simulink model "AMCLIB_FW_BAM"  (Simulink 9.3)
settings: Solver=VariableStepAuto  StartTime=0.0  StopTime=10.0  RelTol=1e-3
settings Model: Creator=nxa18952  LastModifiedBy=nxa18952
settings DataIOCC: SaveFormat=Dataset  SignalLoggingSaveFormat=Dataset  ReturnWorkspaceOutputs=on
settings OptimizationCC: LifeSpan=auto
settings DebuggingCC: UnderspecifiedInitializationDetection=Simplified  MergeDetectMultiDrivingBlocksExec=error  FcnCallInpInsideContextMsg=error  SFUnexpectedBacktrackingDiag=error  SFNoUnconditionalDefaultTransitionDiag=error  SFExecutionAtInitializationDiag=warning  ArithmeticOperatorsInVariantConditions=error
settings HardwareCC: ProdBitPerPointer=64  ProdBitPerSizeT=64  ProdBitPerPtrDiffT=64  ProdLargestAtomicFloat=Float  ProdIntDivRoundTo=Zero  ProdEndianess=LittleEndian  ProdWordSize=64  ProdHWDeviceType=Intel->x86-64 (Windows64)
settings ModelReferenceCC: PropagateSignalLabelsOutOfModel=on
settings SFSimCC: SimUseLocalCustomCode=on
settings RTWCC: RTWUseLocalCustomCode=on
settings CodeAppCC: StateflowObjectComments=off
settings GRTTargetCC: TargetLangStandard=C99 (ISO)  CombineOutputUpdateFcns=on  GRTInterface=off
settings ConfigComp: CovMetricSettings=dwe  CovHtmlReporting=off  CovSaveCumulativeToWorkspaceVar=off  CovSaveSingleToWorkspaceVar=off  CovExternalEMLEnable=on

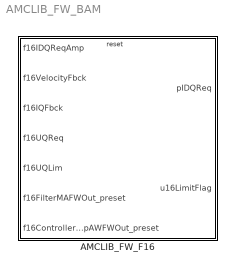
== system AMCLIB_FW_BAM ==
  AMCLIB_FW_F16 : Subsystem  TreatAsAtomicUnit=on  mask(AMCLIB_FW_F16){showStates=Hide (faster execution), resetStatesEnable=Pre-set according to the first set of inputs after reset, showDebugOutputs=Hide, u16NSamples=0, f16PropGain=0, f16IntegGain=0, s16PropGainShift=0, s16IntegGainShift=0, f16LowerLimit=0, f16UpperLimit=0}
      mask prompts: showStates "Show internal states"; resetStatesEnable "Internal state after reset"; showDebugOutputs "Show debugging outputs"; u16NSamples "u16NSamples (GDFLIB_FilterMA - recalculated smoothing factor)"; f16PropGain "f16PropGain (GFLIB_ControllerPIpAW - proportional gain)"; f16IntegGain "f16IntegGain (GFLIB_ControllerPIpAW - integral gain)"; s16PropGainShift "s16PropGainShift (GFLIB_ControllerPIpAW - scaling bitwise shift applied to the proportional gain)"; s16IntegGainShift "s16IntegGainShift (GFLIB_ControllerPIpAW - scaling bitwise shift applied to the integral gain)"; f16LowerLimit "f16LowerLimit (GFLIB_ControllerPIpAW - lower limit)"; f16UpperLimit "f16UpperLimit (GFLIB_ControllerPIpAW - upper limit)"
      mask help: Field Weakening controller for the PMSM field-oriented control algorithm in 16-bit fixed-point fractional implementation. This block supports re-initialization of the internal state during simulation. If the block is reset, the output of the MA filter and PI controller will be aligned with the inputs f16FilterMAFWOut_preset and f16ControllerPIpAWFWOut_preset. Refer to the AMMCLIB User's Guide for further details.
      mask init:
      | if ~evalin('base','exist(''tS8'',''var'')')
      |   if (2 ~= exist('SWLIBS_Typedefs.mat','file'))
      |       error('File SWLIBS_Typedefs.mat is not on the Matlab path. Please add the AMMCLIB "bam" folder in the Matlab Search Path.');
      |   else
      |       evalin('base', 'load(''SWLIBS_Typedefs.mat'')');
      |   end
      | end
      | if showStates == 1
      |     % hidden state variables
      |     if strcmp(get_param([gcb '/u16NSamples'], 'BlockType'), 'Inport')
      |         posblk = get_param(gcb, 'Position');
      | 
      |         pos = get_param(    [gcb, '/u16NSamples'], 'Position');
      |         orient = get_param( [gcb, '/u16NSamples'], 'Orientation');
      |         delete_block(       [gcb, '/u16NSamples']);
      |         add_block('built-in/Ground', [gcb, '/u16NSamples'], 'Position', pos, 'Orientation', orient);
      | 
      |         pos = get_param(    [gcb, '/f16PropGain'], 'Position');
      |         orient = get_param( [gcb, '/f16PropGain'], 'Orientation');
      |         delete_block(       [gcb, '/f16PropGain']);
      |         add_block('built-in/Ground', [gcb, '/f16PropGain'], 'Position', pos, 'Orientation', orient);
      | 
      |         pos = get_param(    [gcb, '/f16IntegGain'], 'Position');
      |         orient = get_param( [gcb, '/f16IntegGain'], 'Orientation');
      |         delete_block(       [gcb, '/f16IntegGain']);
      |         add_block('built-in/Ground', [gcb, '/f16IntegGain'], 'Position', pos, 'Orientation', orient);
      | 
      |         pos = get_param(    [gcb, '/s16PropGainShift'], 'Position');
      |         orient = get_param( [gcb, '/s16PropGainShift'], 'Orientation');
      |         delete_block(       [gcb, '/s16PropGainShift']);
      |         add_block('built-in/Ground', [gcb, '/s16PropGainShift'], 'Position', pos, 'Orientation', orient);
      | 
      |         pos = get_param(    [gcb, '/s16IntegGainShift'], 'Position');
      |         orient = get_param( [gcb, '/s16IntegGainShift'], 'Orientation');
      |         delete_block(       [gcb, '/s16IntegGainShift']);
      |         add_block('built-in/Ground', [gcb, '/s16IntegGainShift'], 'Position', pos, 'Orientation', orient);
      | 
      |         pos = get_param(    [gcb, '/f16LowerLimit'], 'Position');
      |         orient = get_param( [gcb, '/f16LowerLimit'], 'Orientation');
      |         delete_block(       [gcb, '/f16LowerLimit']);
      |         add_block('built-in/Ground', [gcb, '/f16LowerLimit'], 'Position', pos, 'Orientation', orient);
      | 
      |         pos = get_param(    [gcb, '/f16UpperLimit'], 'Position');
      |         orient = get_param( [gcb, '/f16UpperLimit'], 'Orientation');
      |         delete_block(       [gcb, '/f16UpperLimit']);
      |         add_block('built-in/Ground', [gcb, '/f16UpperLimit'], 'Position', pos, 'Orientation', orient);
      | 
      |         pos = get_param(    [gcb, '/f16IQReqK_1'], 'Position');
      |         orient = get_param( [gcb, '/f16IQReqK_1'], 'Orientation');
      |         delete_block(       [gcb, '/f16IQReqK_1']);
      |         add_block('built-in/Ground', [gcb, '/f16IQReqK_1'], 'Position', pos, 'Orientation', orient);
      | 
      |         pos = get_param(    [gcb, '/f32Acc'], 'Position');
      |         orient = get_param( [gcb, '/f32Acc'], 'Orientation');
      |         delete_block(       [gcb, '/f32Acc']);
      |         add_block('built-in/Ground', [gcb, '/f32Acc'], 'Position', pos, 'Orientation', orient);
      | 
      |         pos = get_param(    [gcb, '/f32IntegPartK_1'], 'Position');
      |         orient = get_param( [gcb, '/f32IntegPartK_1'], 'Orientation');
      |         delete_block(       [gcb, '/f32IntegPartK_1']);
      |         add_block('built-in/Ground', [gcb, '/f32IntegPartK_1'], 'Position', pos, 'Orientation', orient);
      | 
      |         pos = get_param(    [gcb, '/f16InK_1'], 'Position');
      |         orient = get_param( [gcb, '/f16InK_1'], 'Orientation');
      |         delete_block(       [gcb, '/f16InK_1']);
      |         add_block('built-in/Ground', [gcb, '/f16InK_1'], 'Position', pos, 'Orientation', orient);
      | 
      | 
      |         pos = get_param(    [gcb '/f32Acc_Out'], 'Position');
      |         orient = get_param( [gcb '/f32Acc_Out'], 'Orientation');
      |         delete_block(       [gcb '/f32Acc_Out']);
      |         add_block('built-in/Terminator', [gcb '/f32Acc_Out'], 'Position', pos, 'Orientation', orient);
      | 
      |         pos = get_param(    [gcb '/f32IntegPartK_1_Out'], 'Position');
      |         orient = get_param( [gcb '/f32IntegPartK_1_Out'], 'Orientation');
      |         delete_block(       [gcb '/f32IntegPartK_1_Out']);
      |         add_block('built-in/Terminator', [gcb '/f32IntegPartK_1_Out'], 'Position', pos, 'Orientation', orient);
      | 
      |         pos = get_param(    [gcb '/f16InK_1_Out'], 'Position');
      |         orient = get_param( [gcb '/f16InK_1_Out'], 'Orientation');
      |         delete_block(       [gcb '/f16InK_1_Out']);
      |         add_block('built-in/Terminator', [gcb '/f16InK_1_Out'], 'Position', pos, 'Orientation', orient);
      | 
      | 
      |         if strcmp(get_param([gcb '/f16IQErrSign'], 'BlockType'), 'Outport')
      |             pos = get_param(    [gcb '/f16IQErrSign'], 'Position');
      |             orient = get_param( [gcb '/f16IQErrSign'], 'Orientation');
      |             delete_block(       [gcb '/f16IQErrSign']);
      |             add_block('built-in/Terminator', [gcb '/f16IQErrSign'], 'Position', pos, 'Orientation', orient);
      | 
      |             pos = get_param(    [gcb '/f16IQErr'], 'Position');
      |             orient = get_param( [gcb '/f16IQErr'], 'Orientation');
      |             delete_block(       [gcb '/f16IQErr']);
      |             add_block('built-in/Terminator', [gcb '/f16IQErr'], 'Position', pos, 'Orientation', orient);
      | 
      |             pos = get_param(    [gcb '/f16FWErr'], 'Position');
      |             orient = get_param( [gcb '/f16FWErr'], 'Orientation');
      |             delete_block(       [gcb '/f16FWErr']);
      |             add_block('built-in/Terminator', [gcb '/f16FWErr'], 'Position', pos, 'Orientation', orient);
      | 
      |             pos = get_param(    [gcb '/f16UQErr'], 'Position');
      |             orient = get_param( [gcb '/f16UQErr'], 'Orientation');
      |             delete_block(       [gcb '/f16UQErr']);
      |             add_block('built-in/Terminator', [gcb '/f16UQErr'], 'Position', pos, 'Orientation', orient);
      | 
      |             pos = get_param(    [gcb '/f16FWErrFilt'], 'Position');
      |             orient = get_param( [gcb '/f16FWErrFilt'], 'Orientation');
      |             delete_block(       [gcb '/f16FWErrFilt']);
      |             add_block('built-in/Terminator', [gcb '/f16FWErrFilt'], 'Position', pos, 'Orientation', orient);
      | 
      |             pos = get_param(    [gcb '/f16FWAngle'], 'Position');
      |             orient = get_param( [gcb '/f16FWAngle'], 'Orientation');
      |             delete_block(       [gcb '/f16FWAngle']);
      |             add_block('built-in/Terminator', [gcb '/f16FWAngle'], 'Position', pos, 'Orientation', orient);
      | 
      |             pos = get_param(    [gcb '/f16FWSin'], 'Position');
      |             orient = get_param( [gcb '/f16FWSin'], 'Orientation');
      |             delete_block(       [gcb '/f16FWSin']);
      |             add_block('built-in/Terminator', [gcb '/f16FWSin'], 'Position', pos, 'Orientation', orient);
      | 
      |             pos = get_param(    [gcb '/f16FWCos'], 'Position');
      |             orient = get_param( [gcb '/f16FWCos'], 'Orientation');
      |             delete_block(       [gcb '/f16FWCos']);
      |             add_block('built-in/Terminator', [gcb '/f16FWCos'], 'Position', pos, 'Orientation', orient);
      | 
      |         end
      | 
      |         set_param([gcb '/f16IDQReqAmp'], 'Port', '1');
      |         set_param([gcb '/f16VelocityFbck'], 'Port', '2');
      |         set_param([gcb '/f16IQFbck'], 'Port', '3');
      |         set_param([gcb '/f16UQReq'], 'Port', '4');
      |         set_param([gcb '/f16UQLim'], 'Port', '5');
      |         set_param([gcb '/f16FilterMAFWOut_preset'], 'Port', '6');
      |         set_param([gcb '/f16ControllerPIpAWFWOut_preset'], 'Port', '7');
      | 
      |         set_param([gcb '/pIDQReq'], 'Port', '1');
      |         set_param([gcb '/u16LimitFlag'], 'Port', '2');
      | 
      |         set_param(gcb,'MaskEnables',{'on','on','off','on','on','on','on','on','on','on'});
      | 
      |         if (posblk(4) - posblk(2)) > 200
      |           height = 200;
      |           set_param(gcb,'Position',[posblk(1), posblk(2), posblk(3), posblk(2)+height])
      |         end
      |     end
      | else
      |     % shown state variables
      |     if strcmp(get_param([gcb '/u16NSamples'], 'BlockType'), 'Ground')
      |         posblk = get_param(gcb, 'Position');
      | 
      |         pos = get_param(    [gcb, '/u16NSamples'], 'Position');
      |         orient = get_param( [gcb, '/u16NSamples'], 'Orientation');
      |         delete_block(       [gcb, '/u16NSamples']);
      |         add_block('built-in/Inport', [gcb, '/u16NSamples'], 'Position', pos, 'Orientation', orient, 'OutDataTypeStr', 'uint16');
      | 
      |         pos = get_param(    [gcb, '/f16PropGain'], 'Position');
      |         orient = get_param( [gcb, '/f16PropGain'], 'Orientation');
      |         delete_block(       [gcb, '/f16PropGain']);
      |         add_block('built-in/Inport', [gcb, '/f16PropGain'], 'Position', pos, 'Orientation', orient, 'OutDataTypeStr', 'int16');
      | 
      |         pos = get_param(    [gcb, '/f16IntegGain'], 'Position');
      |         orient = get_param( [gcb, '/f16IntegGain'], 'Orientation');
      |         delete_block(       [gcb, '/f16IntegGain']);
      |         add_block('built-in/Inport', [gcb, '/f16IntegGain'], 'Position', pos, 'Orientation', orient, 'OutDataTypeStr', 'int16');
      | 
      |         pos = get_param(    [gcb, '/s16PropGainShift'], 'Position');
      |         orient = get_param( [gcb, '/s16PropGainShift'], 'Orientation');
      |         delete_block(       [gcb, '/s16PropGainShift']);
      |         add_block('built-in/Inport', [gcb, '/s16PropGainShift'], 'Position', pos, 'Orientation', orient, 'OutDataTypeStr', 'int16');
      | 
      |         pos = get_param(    [gcb, '/s16IntegGainShift'], 'Position');
      |         orient = get_param( [gcb, '/s16IntegGainShift'], 'Orientation');
      |         delete_block(       [gcb, '/s16IntegGainShift']);
      |         add_block('built-in/Inport', [gcb, '/s16IntegGainShift'], 'Position', pos, 'Orientation', orient, 'OutDataTypeStr', 'int16');
      | 
      |         pos = get_param(    [gcb, '/f16LowerLimit'], 'Position');
      |         orient = get_param( [gcb, '/f16LowerLimit'], 'Orientation');
      |         delete_block(       [gcb, '/f16LowerLimit']);
      |         add_block('built-in/Inport', [gcb, '/f16LowerLimit'], 'Position', pos, 'Orientation', orient, 'OutDataTypeStr', 'int16');
      | 
      |         pos = get_param(    [gcb, '/f16UpperLimit'], 'Position');
      |         orient = get_param( [gcb, '/f16UpperLimit'], 'Orientation');
      |         delete_block(       [gcb, '/f16UpperLimit']);
      |         add_block('built-in/Inport', [gcb, '/f16UpperLimit'], 'Position', pos, 'Orientation', orient, 'OutDataTypeStr', 'int16');
      | 
      |         pos = get_param(    [gcb, '/f16IQReqK_1'], 'Position');
      |         orient = get_param( [gcb, '/f16IQReqK_1'], 'Orientation');
      |         delete_block(       [gcb, '/f16IQReqK_1']);
      |         add_block('built-in/Inport', [gcb, '/f16IQReqK_1'], 'Position', pos, 'Orientation', orient, 'OutDataTypeStr', 'int16');
      | 
      |         pos = get_param(    [gcb, '/f32Acc'], 'Position');
      |         orient = get_param( [gcb, '/f32Acc'], 'Orientation');
      |         delete_block(       [gcb, '/f32Acc']);
      |         add_block('built-in/Inport', [gcb, '/f32Acc'], 'Position', pos, 'Orientation', orient, 'OutDataTypeStr', 'int32');
      | 
      |         pos = get_param(    [gcb, '/f32IntegPartK_1'], 'Position');
      |         orient = get_param( [gcb, '/f32IntegPartK_1'], 'Orientation');
      |         delete_block(       [gcb, '/f32IntegPartK_1']);
      |         add_block('built-in/Inport', [gcb, '/f32IntegPartK_1'], 'Position', pos, 'Orientation', orient, 'OutDataTypeStr', 'int32');
      | 
      |         pos = get_param(    [gcb, '/f16InK_1'], 'Position');
      |         orient = get_param( [gcb, '/f16InK_1'], 'Orientation');
      |         delete_block(       [gcb, '/f16InK_1']);
      |         add_block('built-in/Inport', [gcb, '/f16InK_1'], 'Position', pos, 'Orientation', orient, 'OutDataTypeStr', 'int16');
      | 
      | 
      |         pos = get_param(    [gcb '/f32Acc_Out'], 'Position');
      |         orient = get_param( [gcb '/f32Acc_Out'], 'Orientation');
      |         delete_block(       [gcb '/f32Acc_Out']);
      |         add_block('built-in/Outport', [gcb '/f32Acc_Out'], 'Position', pos, 'Orientation', orient);
      | 
      |         pos = get_param(    [gcb '/f32IntegPartK_1_Out'], 'Position');
      |         orient = get_param( [gcb '/f32IntegPartK_1_Out'], 'Orientation');
      |         delete_block(       [gcb '/f32IntegPartK_1_Out']);
      |         add_block('built-in/Outport', [gcb '/f32IntegPartK_1_Out'], 'Position', pos, 'Orientation', orient);
      | 
      |         pos = get_param(    [gcb '/f16InK_1_Out'], 'Position');
      |         orient = get_param( [gcb '/f16InK_1_Out'], 'Orientation');
      |         delete_block(       [gcb '/f16InK_1_Out']);
      |         add_block('built-in/Outport', [gcb '/f16InK_1_Out'], 'Position', pos, 'Orientation', orient);
      | 
      | 
      |         if (showDebugOutputs == 2) && (strcmp(get_param([gcb '/f16IQErrSign'], 'BlockType'), 'Terminator'))
      |             pos = get_param(    [gcb '/f16IQErrSign'], 'Position');
      |             orient = get_param( [gcb '/f16IQErrSign'], 'Orientation');
      |             delete_block(       [gcb '/f16IQErrSign']);
      |             add_block('built-in/Outport', [gcb '/f16IQErrSign'], 'Position', pos, 'Orientation', orient);
      | 
      |             pos = get_param(    [gcb '/f16IQErr'], 'Position');
      |             orient = get_param( [gcb '/f16IQErr'], 'Orientation');
      |             delete_block(       [gcb '/f16IQErr']);
      |             add_block('built-in/Outport', [gcb '/f16IQErr'], 'Position', pos, 'Orientation', orient);
      | 
      |             pos = get_param(    [gcb '/f16FWErr'], 'Position');
      |             orient = get_param( [gcb '/f16FWErr'], 'Orientation');
      |             delete_block(       [gcb '/f16FWErr']);
      |             add_block('built-in/Outport', [gcb '/f16FWErr'], 'Position', pos, 'Orientation', orient);
      | 
      |             pos = get_param(    [gcb '/f16UQErr'], 'Position');
      |             orient = get_param( [gcb '/f16UQErr'], 'Orientation');
      |             delete_block(       [gcb '/f16UQErr']);
      |             add_block('built-in/Outport', [gcb '/f16UQErr'], 'Position', pos, 'Orientation', orient);
      | 
      |             pos = get_param(    [gcb '/f16FWErrFilt'], 'Position');
      |             orient = get_param( [gcb '/f16FWErrFilt'], 'Orientation');
      |             delete_block(       [gcb '/f16FWErrFilt']);
      |             add_block('built-in/Outport', [gcb '/f16FWErrFilt'], 'Position', pos, 'Orientation', orient);
      | 
      |             pos = get_param(    [gcb '/f16FWAngle'], 'Position');
      |             orient = get_param( [gcb '/f16FWAngle'], 'Orientation');
      |             delete_block(       [gcb '/f16FWAngle']);
      |             add_block('built-in/Outport', [gcb '/f16FWAngle'], 'Position', pos, 'Orientation', orient);
      | 
      |             pos = get_param(    [gcb '/f16FWSin'], 'Position');
      |             orient = get_param( [gcb '/f16FWSin'], 'Orientation');
      |             delete_block(       [gcb '/f16FWSin']);
      |             add_block('built-in/Outport', [gcb '/f16FWSin'], 'Position', pos, 'Orientation', orient);
      | 
      |             pos = get_param(    [gcb '/f16FWCos'], 'Position');
      |             orient = get_param( [gcb '/f16FWCos'], 'Orientation');
      |             delete_block(       [gcb '/f16FWCos']);
      |             add_block('built-in/Outport', [gcb '/f16FWCos'], 'Position', pos, 'Orientation', orient);
      | 
      |         end
      | 
      |         set_param([gcb '/f16IDQReqAmp'], 'Port', '1');
      |         set_param([gcb '/f16VelocityFbck'], 'Port', '2');
      |         set_param([gcb '/f16IQFbck'], 'Port', '3');
      |         set_param([gcb '/f16UQReq'], 'Port', '4');
      |         set_param([gcb '/f16UQLim'], 'Port', '5');
      |         set_param([gcb '/f16FilterMAFWOut_preset'], 'Port', '6');
      |         set_param([gcb '/f16ControllerPIpAWFWOut_preset'], 'Port', '7');
      |         set_param([gcb '/u16NSamples'], 'Port', '8');
      |         set_param([gcb '/f16PropGain'], 'Port', '9');
      |         set_param([gcb '/f16IntegGain'], 'Port', '10');
      |         set_param([gcb '/s16PropGainShift'], 'Port', '11');
      |         set_param([gcb '/s16IntegGainShift'], 'Port', '12');
      |         set_param([gcb '/f16LowerLimit'], 'Port', '13');
      |         set_param([gcb '/f16UpperLimit'], 'Port', '14');
      |         set_param([gcb '/f16IQReqK_1'], 'Port', '15');
      |         set_param([gcb '/f32Acc'], 'Port', '16');
      |         set_param([gcb '/f32IntegPartK_1'], 'Port', '17');
      |         set_param([gcb '/f16InK_1'], 'Port', '18');
      | 
      |         if (showDebugOutputs == 2)
      |             set_param([gcb '/pIDQReq'], 'Port', '1');
      |             set_param([gcb '/u16LimitFlag'], 'Port', '2');
      |             set_param([gcb '/f16IQErrSign'], 'Port', '3');
      |             set_param([gcb '/f16IQErr'], 'Port', '4');
      |             set_param([gcb '/f16FWErr'], 'Port', '5');
      |             set_param([gcb '/f16UQErr'], 'Port', '6');
      |             set_param([gcb '/f16FWErrFilt'], 'Port', '7');
      |             set_param([gcb '/f16FWAngle'], 'Port', '8');
      |             set_param([gcb '/f16FWSin'], 'Port', '9');
      |             set_param([gcb '/f16FWCos'], 'Port', '10');
      |             set_param([gcb '/f32Acc_Out'], 'Port', '11');
      |             set_param([gcb '/f32IntegPartK_1_Out'], 'Port', '12');
      |             set_param([gcb '/f16InK_1_Out'], 'Port', '13');
      |         else
      |             set_param([gcb '/pIDQReq'], 'Port', '1');
      |             set_param([gcb '/u16LimitFlag'], 'Port', '2');
      |             set_param([gcb '/f32Acc_Out'], 'Port', '3');
      |             set_param([gcb '/f32IntegPartK_1_Out'], 'Port', '4');
      |             set_param([gcb '/f16InK_1_Out'], 'Port', '5');
      |         end
      | 
      |         set_param(gcb,'MaskEnables',{'on','on','on','off','off','off','off','off','off','off'});
      | 
      |         if (posblk(4) - posblk(2)) < 475
      |           height = 475;
      |           set_param(gcb,'Position',[posblk(1), posblk(2), posblk(3), posblk(2)+height])
      |         end
      |     else
      |         if (showDebugOutputs == 2) && (strcmp(get_param([gcb '/f16IQErrSign'], 'BlockType'), 'Terminator'))
      |             % shown debugging outputs
      |             pos = get_param(    [gcb '/f16IQErrSign'], 'Position');
      |             orient = get_param( [gcb '/f16IQErrSign'], 'Orientation');
      |             delete_block(       [gcb '/f16IQErrSign']);
      |             add_block('built-in/Outport', [gcb '/f16IQErrSign'], 'Position', pos, 'Orientation', orient);
      | 
      |             pos = get_param(    [gcb '/f16IQErr'], 'Position');
      |             orient = get_param( [gcb '/f16IQErr'], 'Orientation');
      |             delete_block(       [gcb '/f16IQErr']);
      |             add_block('built-in/Outport', [gcb '/f16IQErr'], 'Position', pos, 'Orientation', orient);
      | 
      |             pos = get_param(    [gcb '/f16FWErr'], 'Position');
      |             orient = get_param( [gcb '/f16FWErr'], 'Orientation');
      |             delete_block(       [gcb '/f16FWErr']);
      |             add_block('built-in/Outport', [gcb '/f16FWErr'], 'Position', pos, 'Orientation', orient);
      | 
      |             pos = get_param(    [gcb '/f16UQErr'], 'Position');
      |             orient = get_param( [gcb '/f16UQErr'], 'Orientation');
      |             delete_block(       [gcb '/f16UQErr']);
      |             add_block('built-in/Outport', [gcb '/f16UQErr'], 'Position', pos, 'Orientation', orient);
      | 
      |             pos = get_param(    [gcb '/f16FWErrFilt'], 'Position');
      |             orient = get_param( [gcb '/f16FWErrFilt'], 'Orientation');
      |             delete_block(       [gcb '/f16FWErrFilt']);
      |             add_block('built-in/Outport', [gcb '/f16FWErrFilt'], 'Position', pos, 'Orientation', orient);
      | 
      |             pos = get_param(    [gcb '/f16FWAngle'], 'Position');
      |             orient = get_param( [gcb '/f16FWAngle'], 'Orientation');
      |             delete_block(       [gcb '/f16FWAngle']);
      |             add_block('built-in/Outport', [gcb '/f16FWAngle'], 'Position', pos, 'Orientation', orient);
      | 
      |             pos = get_param(    [gcb '/f16FWSin'], 'Position');
      |             orient = get_param( [gcb '/f16FWSin'], 'Orientation');
      |             delete_block(       [gcb '/f16FWSin']);
      |             add_block('built-in/Outport', [gcb '/f16FWSin'], 'Position', pos, 'Orientation', orient);
      | 
      |             pos = get_param(    [gcb '/f16FWCos'], 'Position');
      |             orient = get_param( [gcb '/f16FWCos'], 'Orientation');
      |             delete_block(       [gcb '/f16FWCos']);
      |             add_block('built-in/Outport', [gcb '/f16FWCos'], 'Position', pos, 'Orientation', orient);
      | 
      |             set_param([gcb '/pIDQReq'], 'Port', '1');
      |             set_param([gcb '/u16LimitFlag'], 'Port', '2');
      |             set_param([gcb '/f16IQErrSign'], 'Port', '3');
      |             set_param([gcb '/f16IQErr'], 'Port', '4');
      |             set_param([gcb '/f16FWErr'], 'Port', '5');
      |             set_param([gcb '/f16UQErr'], 'Port', '6');
      |             set_param([gcb '/f16FWErrFilt'], 'Port', '7');
      |             set_param([gcb '/f16FWAngle'], 'Port', '8');
      |             set_param([gcb '/f16FWSin'], 'Port', '9');
      |             set_param([gcb '/f16FWCos'], 'Port', '10');
      |             set_param([gcb '/f32Acc_Out'], 'Port', '11');
      |             set_param([gcb '/f32IntegPartK_1_Out'], 'Port', '12');
      |             set_param([gcb '/f16InK_1_Out'], 'Port', '13');
      |         elseif (showDebugOutputs == 1) && (strcmp(get_param([gcb '/f16IQErrSign'], 'BlockType'), 'Outport'))
      |             % hidden debugging outputs
      |             pos = get_param(    [gcb '/f16IQErrSign'], 'Position');
      |             orient = get_param( [gcb '/f16IQErrSign'], 'Orientation');
      |             delete_block(       [gcb '/f16IQErrSign']);
      |             add_block('built-in/Terminator', [gcb '/f16IQErrSign'], 'Position', pos, 'Orientation', orient);
      | 
      |             pos = get_param(    [gcb '/f16IQErr'], 'Position');
      |             orient = get_param( [gcb '/f16IQErr'], 'Orientation');
      |             delete_block(       [gcb '/f16IQErr']);
      |             add_block('built-in/Terminator', [gcb '/f16IQErr'], 'Position', pos, 'Orientation', orient);
      | 
      |             pos = get_param(    [gcb '/f16FWErr'], 'Position');
      |             orient = get_param( [gcb '/f16FWErr'], 'Orientation');
      |             delete_block(       [gcb '/f16FWErr']);
      |             add_block('built-in/Terminator', [gcb '/f16FWErr'], 'Position', pos, 'Orientation', orient);
      | 
      |             pos = get_param(    [gcb '/f16UQErr'], 'Position');
      |             orient = get_param( [gcb '/f16UQErr'], 'Orientation');
      |             delete_block(       [gcb '/f16UQErr']);
      |             add_block('built-in/Terminator', [gcb '/f16UQErr'], 'Position', pos, 'Orientation', orient);
      | 
      |             pos = get_param(    [gcb '/f16FWErrFilt'], 'Position');
      |             orient = get_param( [gcb '/f16FWErrFilt'], 'Orientation');
      |             delete_block(       [gcb '/f16FWErrFilt']);
      |             add_block('built-in/Terminator', [gcb '/f16FWErrFilt'], 'Position', pos, 'Orientation', orient);
      | 
      |             pos = get_param(    [gcb '/f16FWAngle'], 'Position');
      |             orient = get_param( [gcb '/f16FWAngle'], 'Orientation');
      |             delete_block(       [gcb '/f16FWAngle']);
      |             add_block('built-in/Terminator', [gcb '/f16FWAngle'], 'Position', pos, 'Orientation', orient);
      | 
      |             pos = get_param(    [gcb '/f16FWSin'], 'Position');
      |             orient = get_param( [gcb '/f16FWSin'], 'Orientation');
      |             delete_block(       [gcb '/f16FWSin']);
      |             add_block('built-in/Terminator', [gcb '/f16FWSin'], 'Position', pos, 'Orientation', orient);
      | 
      |             pos = get_param(    [gcb '/f16FWCos'], 'Position');
      |             orient = get_param( [gcb '/f16FWCos'], 'Orientation');
      |             delete_block(       [gcb '/f16FWCos']);
      |             add_block('built-in/Terminator', [gcb '/f16FWCos'], 'Position', pos, 'Orientation', orient);
      | 
      |             set_param([gcb '/pIDQReq'], 'Port', '1');
      |             set_param([gcb '/u16LimitFlag'], 'Port', '2');
      |             set_param([gcb '/f32Acc_Out'], 'Port', '3');
      |             set_param([gcb '/f32IntegPartK_1_Out'], 'Port', '4');
      |             set_param([gcb '/f16InK_1_Out'], 'Port', '5');
      |         end
      |     end
      | end
      settings: RTWSystemCode=Inline
      mask TypeOptions showStates: Hide (faster execution) | Show (allows debugging; connect feedback loops manually)
      mask Callback showStates:
      | maskStr = get_param(gcb,'showStates');
      | if strcmp(maskStr,'Hide (faster execution)'),
      |     set_param(gcb,'MaskEnables',{'on','on','off','on','on','on','on','on','on','on'});
      | else
      |     set_param(gcb,'MaskEnables',{'on','on','on','off','off','off','off','off','off','off'});
      | end
      mask TypeOptions resetStatesEnable: Pre-set according to the first set of inputs after reset | Clear to zero
      mask TypeOptions showDebugOutputs: Hide | Show
      mask Display:
      | color('black');
      | pos = get_param(gcb, 'Position');
      | width = pos(3) - pos(1);
      | height = pos(4) - pos(2);
      | tX=width/2;
      | tY=height - 25;
      | color('black');
      | text(tX,tY, 'AMCLIB_FW_F16', 'horizontalAlignment', 'center');
      | if showStates == 2
      |   color('red');
      |   text(tX,tY - 20, ['debugging mode' char(13) char(10) '(limited performance)'], 'horizontalAlignment', 'center');
      | end

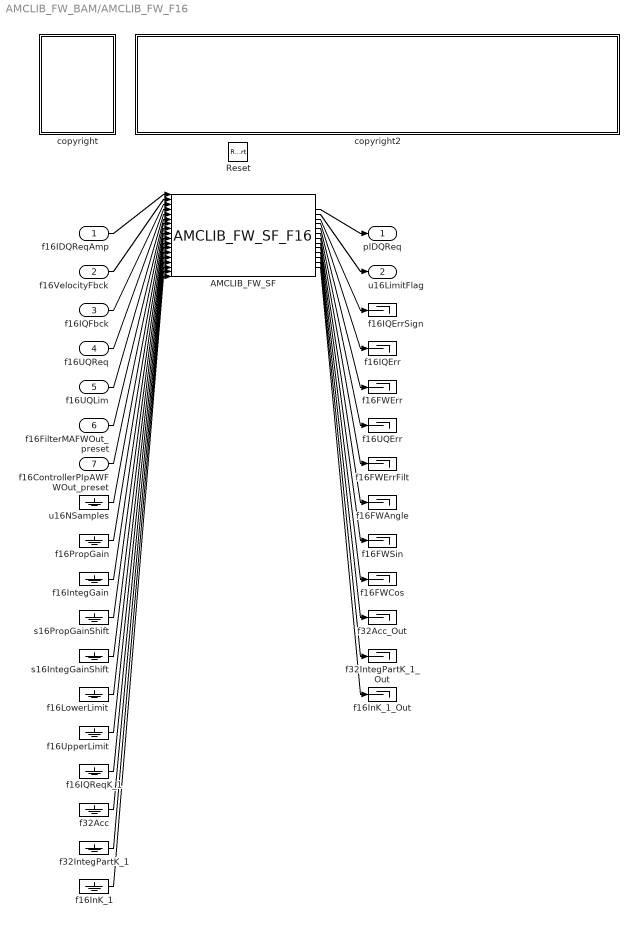
== system AMCLIB_FW_BAM/AMCLIB_FW_F16 ==
  f16IDQReqAmp : Inport  OutDataTypeStr=int16
  f16VelocityFbck : Inport  Port=2  OutDataTypeStr=int16
  f16IQFbck : Inport  Port=3  OutDataTypeStr=int16
  f16UQReq : Inport  Port=4  OutDataTypeStr=int16
  f16UQLim : Inport  Port=5  OutDataTypeStr=int16
  f16FilterMAFWOut_preset : Inport  Port=6  OutDataTypeStr=int16
  f16ControllerPIpAWFWOut_preset : Inport  Port=7  OutDataTypeStr=int16
  Reset : ResetPort  DisableCoverage=on
  AMCLIB_FW_SF : S-Function  FunctionName=AMCLIB_FW_SF_F16  Parameters=showStates,resetStatesEnable,showDebugOutputs,u16NSamples,f16PropGain,f16IntegGain,s16PropGainShift,s16IntegGainShift,f16LowerLimit,f16UpperLimit  SFunctionDeploymentMode=off  EnableBusSupport=off
  copyright : Subsystem
      mask Display: text(10,90,'FILE:');text(10,75,'DESRIPTION:');text(10,60,'COPYRIGHT:');text(10,45,'VERSION:');text(10,30,'DATE:')
  copyright2 : Subsystem
      mask Display: text(10,90,'AMCLIB_FW_BAM_F16.mdl');text(10,75,'PMSM Field Weakening Controller');text(10,60,'NXP 2020');text(10,45,'1.0');text(10,30,'28-Mar-2020');
  f16FWAngle : Terminator
  f16FWCos : Terminator
  f16FWErr : Terminator
  f16FWErrFilt : Terminator
  f16FWSin : Terminator
  f16IQErr : Terminator
  f16IQErrSign : Terminator
  f16IQReqK_1 : Ground
  f16InK_1 : Ground
  f16InK_1_Out : Terminator
  f16IntegGain : Ground
  f16LowerLimit : Ground
  f16PropGain : Ground
  f16UQErr : Terminator
  f16UpperLimit : Ground
  f32Acc : Ground
  f32Acc_Out : Terminator
  f32IntegPartK_1 : Ground
  f32IntegPartK_1_Out : Terminator
  s16IntegGainShift : Ground
  s16PropGainShift : Ground
  u16NSamples : Ground
  pIDQReq : Outport
  u16LimitFlag : Outport  Port=2
  wires:
  f16IDQReqAmp/1 -> AMCLIB_FW_SF/1
  f16VelocityFbck/1 -> AMCLIB_FW_SF/2
  f16IQFbck/1 -> AMCLIB_FW_SF/3
  f16UQReq/1 -> AMCLIB_FW_SF/4
  f16UQLim/1 -> AMCLIB_FW_SF/5
  f16FilterMAFWOut_preset/1 -> AMCLIB_FW_SF/6
  f16ControllerPIpAWFWOut_preset/1 -> AMCLIB_FW_SF/7
  u16NSamples/1 -> AMCLIB_FW_SF/8
  f16PropGain/1 -> AMCLIB_FW_SF/9
  f16IntegGain/1 -> AMCLIB_FW_SF/10
  s16PropGainShift/1 -> AMCLIB_FW_SF/11
  s16IntegGainShift/1 -> AMCLIB_FW_SF/12
  f16LowerLimit/1 -> AMCLIB_FW_SF/13
  f16UpperLimit/1 -> AMCLIB_FW_SF/14
  f16IQReqK_1/1 -> AMCLIB_FW_SF/15
  f32Acc/1 -> AMCLIB_FW_SF/16
  f32IntegPartK_1/1 -> AMCLIB_FW_SF/17
  f16InK_1/1 -> AMCLIB_FW_SF/18
  AMCLIB_FW_SF/1 -> pIDQReq/1
  AMCLIB_FW_SF/2 -> u16LimitFlag/1
  AMCLIB_FW_SF/3 -> f16IQErrSign/1
  AMCLIB_FW_SF/4 -> f16IQErr/1
  AMCLIB_FW_SF/5 -> f16FWErr/1
  AMCLIB_FW_SF/6 -> f16UQErr/1
  AMCLIB_FW_SF/7 -> f16FWErrFilt/1
  AMCLIB_FW_SF/8 -> f16FWAngle/1
  AMCLIB_FW_SF/9 -> f16FWSin/1
  AMCLIB_FW_SF/10 -> f16FWCos/1
  AMCLIB_FW_SF/11 -> f32Acc_Out/1
  AMCLIB_FW_SF/12 -> f32IntegPartK_1_Out/1
  AMCLIB_FW_SF/13 -> f16InK_1_Out/1

== system AMCLIB_FW_BAM/AMCLIB_FW_F16/copyright ==

== system AMCLIB_FW_BAM/AMCLIB_FW_F16/copyright2 ==
